simulink library "simulink"  (Simulink 6.0)
settings: Solver=ode45  SolverMode=SingleTasking  StartTime=0.0  StopTime=10.0  RelTol=1e-3
PostLoadFcn:
  | setsysloc(bdroot)
undefined symbols (not defined in the file or in its folder): DiscIntNeverNeededParam, getdatatypespecs, NumBits1, NumBits2, sfunxy, sigbuilder_block, slcm, Slope1, Slope2
libraries: simulink x82, eml_lib x1
(part 4 of 5)

== system simulink/Model Verification/Check  Dynamic Gap ==
  max : Inport  LatchInput=off
  min : Inport  Port=2  LatchInput=off
  u : Inport  Port=3  LatchInput=off
  Assertion : Assertion
      settings: CopyFcn=set_param(gcbh,'ShadowObject',get_param(get_param(gcbh,'Parent'),'Handle'));
  disjunction : Logic  Operator=OR
  max_relop : RelationalOperator  Operator=<  InputSameDT=on
  maxtype : DataTypeConversion  SaturateOnIntegerOverflow=on  RndMeth=Zero
  min_relop : RelationalOperator  Operator=<  InputSameDT=on
  mintype : DataTypeConversion  SaturateOnIntegerOverflow=on  RndMeth=Zero
  out : Terminator
  wires:
  max/1 -> maxtype/1
  min/1 -> mintype/1
  u/1 -> min_relop/1, max_relop/2
  disjunction/1 -> Assertion/1, out/1
  min_relop/1 -> disjunction/2
  max_relop/1 -> disjunction/1
  mintype/1 -> min_relop/2
  maxtype/1 -> max_relop/1

== system simulink/Model Verification/Check  Dynamic Range ==
  max : Inport  LatchInput=off
  min : Inport  Port=2  LatchInput=off
  u : Inport  Port=3  LatchInput=off
  Assertion : Assertion
      settings: CopyFcn=set_param(gcbh,'ShadowObject',get_param(get_param(gcbh,'Parent'),'Handle'));
  conjunction : Logic
  max_relop : RelationalOperator  Operator=<  InputSameDT=on
  maxtype : DataTypeConversion  SaturateOnIntegerOverflow=on  RndMeth=Zero
  min_relop : RelationalOperator  Operator=<  InputSameDT=on
  mintype : DataTypeConversion  SaturateOnIntegerOverflow=on  RndMeth=Zero
  out : Terminator
  wires:
  u/1 -> max_relop/1, min_relop/2
  min/1 -> mintype/1
  mintype/1 -> min_relop/1
  max/1 -> maxtype/1
  maxtype/1 -> max_relop/2
  min_relop/1 -> conjunction/1
  max_relop/1 -> conjunction/2
  conjunction/1 -> Assertion/1, out/1

== system simulink/Model Verification/Check  Static Gap ==
  u : Inport  LatchInput=off
  Assertion : Assertion
      settings: CopyFcn=set_param(gcbh,'ShadowObject',get_param(get_param(gcbh,'Parent'),'Handle'));
  disjunction : Logic  Operator=OR
  max_relop : RelationalOperator  Operator=<=  InputSameDT=on
  max_val : Constant  Value=max
  maxtype : DataTypeConversion  SaturateOnIntegerOverflow=on  RndMeth=Zero
  min_relop : RelationalOperator  Operator=<=  InputSameDT=on
  min_val : Constant  Value=min
  mintype : DataTypeConversion  SaturateOnIntegerOverflow=on  RndMeth=Zero
  out : Terminator
  wires:
  mintype/1 -> min_relop/2
  maxtype/1 -> max_relop/1
  min_val/1 -> mintype/1
  max_val/1 -> maxtype/1
  u/1 -> max_relop/2, min_relop/1
  max_relop/1 -> disjunction/1
  min_relop/1 -> disjunction/2
  disjunction/1 -> Assertion/1, out/1

== system simulink/Model Verification/Check  Static Range ==
  u : Inport  LatchInput=off
  Assertion : Assertion
      settings: CopyFcn=set_param(gcbh,'ShadowObject',get_param(get_param(gcbh,'Parent'),'Handle'));
  conjunction : Logic
  max_relop : RelationalOperator  Operator=<=  InputSameDT=on
  max_val : Constant  Value=max
  maxtype : DataTypeConversion  SaturateOnIntegerOverflow=on  RndMeth=Zero
  min_relop : RelationalOperator  Operator=<=  InputSameDT=on
  min_val : Constant  Value=min
  mintype : DataTypeConversion  SaturateOnIntegerOverflow=on  RndMeth=Zero
  out : Terminator
  wires:
  maxtype/1 -> max_relop/2
  mintype/1 -> min_relop/1
  conjunction/1 -> Assertion/1, out/1
  max_relop/1 -> conjunction/2
  min_relop/1 -> conjunction/1
  max_val/1 -> maxtype/1
  min_val/1 -> mintype/1
  u/1 -> max_relop/1, min_relop/2

== system simulink/Model Verification/Check Dynamic  Lower Bound ==
  min : Inport  LatchInput=off
  u : Inport  Port=2  LatchInput=off
  Assertion : Assertion
      settings: CopyFcn=set_param(gcbh,'ShadowObject',get_param(get_param(gcbh,'Parent'),'Handle'));
  min_relop : RelationalOperator  Operator=<  InputSameDT=on
  mintype : DataTypeConversion  SaturateOnIntegerOverflow=on  RndMeth=Zero
  out : Terminator
  wires:
  u/1 -> min_relop/2
  mintype/1 -> min_relop/1
  min/1 -> mintype/1
  min_relop/1 -> Assertion/1, out/1

== system simulink/Model Verification/Check Dynamic  Upper Bound ==
  max : Inport  LatchInput=off
  u : Inport  Port=2  LatchInput=off
  Assertion : Assertion
      settings: CopyFcn=set_param(gcbh,'ShadowObject',get_param(get_param(gcbh,'Parent'),'Handle'));
  max_relop : RelationalOperator  Operator=<  InputSameDT=on
  maxtype : DataTypeConversion  SaturateOnIntegerOverflow=on  RndMeth=Zero
  out : Terminator
  wires:
  u/1 -> max_relop/1
  max/1 -> maxtype/1
  maxtype/1 -> max_relop/2
  max_relop/1 -> Assertion/1, out/1

== system simulink/Model Verification/Check Input  Resolution ==
  u : Inport  LatchInput=off
  Assertion : Assertion
      settings: CopyFcn=set_param(gcbh,'ShadowObject',get_param(get_param(gcbh,'Parent'),'Handle'));
  dead_out : Terminator
  dead_resolution : Constant  Value=[1 1]
  dead_u : Constant
  fixed : Subsystem
  out : Terminator
  resolution : Constant  Value=resolution
  resolution_type : DataTypeConversion  SaturateOnIntegerOverflow=on  RndMeth=Zero
  steps : Subsystem
  wires:
  resolution/1 -> resolution_type/1
  u/1 -> steps/1(u)
  resolution_type/1 -> steps/2(resolution)
  steps/1(out) -> Assertion/1, out/1
  dead_u/1 -> fixed/1(u)
  dead_resolution/1 -> fixed/2(resolution)
  fixed/1(out) -> dead_out/1

== system simulink/Model Verification/Check Static  Lower Bound ==
  u : Inport  LatchInput=off
  Assertion : Assertion
      settings: CopyFcn=set_param(gcbh,'ShadowObject',get_param(get_param(gcbh,'Parent'),'Handle'));
  min_relop : RelationalOperator  Operator=<=  InputSameDT=on
  min_val : Constant  Value=min
  mintype : DataTypeConversion  SaturateOnIntegerOverflow=on  RndMeth=Zero
  out : Terminator
  wires:
  min_relop/1 -> Assertion/1, out/1
  u/1 -> min_relop/2
  min_val/1 -> mintype/1
  mintype/1 -> min_relop/1

== system simulink/Model Verification/Check Static  Upper Bound ==
  u : Inport  LatchInput=off
  Assertion : Assertion
      settings: CopyFcn=set_param(gcbh,'ShadowObject',get_param(get_param(gcbh,'Parent'),'Handle'));
  max_relop : RelationalOperator  Operator=<=  InputSameDT=on
  max_val : Constant  Value=max
  mintype : DataTypeConversion  SaturateOnIntegerOverflow=on  RndMeth=Zero
  out : Terminator
  wires:
  mintype/1 -> max_relop/2
  u/1 -> max_relop/1
  max_val/1 -> mintype/1
  max_relop/1 -> Assertion/1, out/1

== system simulink/Model-Wide Utilities/Block Support Table ==
  EmptySubsystem : Subsystem

== system simulink/Model-Wide Utilities/DocBlock ==
  EmptySubsystem : Subsystem

== system simulink/Model-Wide Utilities/Model Info ==
  EmptySubsystem : Subsystem

== system simulink/Model-Wide Utilities/Timed-Based Linearization ==
  Clock : Clock
      settings: Decimation=10
  Constant : Constant  Value=LinearizationTime
  Sum : Sum  Inputs=-+  SaturateOnIntegerOverflow=on  InputSameDT=on
  Triggered Linearization : Subsystem  Orientation=down  TreatAsAtomicUnit=on
  wires:
  Clock/1 -> Sum/2
  Constant/1 -> Sum/1
  Sum/1 -> Triggered Linearization/Trigger

== system simulink/Model-Wide Utilities/Trigger-Based Linearization ==
  Trigger : TriggerPort
  S-Function : S-Function  FunctionName=sfunlin  Parameters=name_,SampleTime

== system simulink/Ports & Subsystems/Atomic Subsystem ==
  In1 : Inport  LatchInput=off
  Out1 : Outport
  wires:
  In1/1 -> Out1/1

== system simulink/Ports & Subsystems/CodeReuseSubsystem ==
  In1 : Inport  LatchInput=off
  Out1 : Outport
  wires:
  In1/1 -> Out1/1

== system simulink/Ports & Subsystems/Configurable Subsystem ==

== system simulink/Ports & Subsystems/Enabled Subsystem ==
  In1 : Inport  LatchInput=off
  Enable : EnablePort
  Out1 : Outport
  wires:
  In1/1 -> Out1/1

== system simulink/Ports & Subsystems/Enabled and Triggered Subsystem ==
  In1 : Inport  LatchInput=off
  Enable : EnablePort
  Trigger : TriggerPort
  Out1 : Outport
  wires:
  In1/1 -> Out1/1

== system simulink/Ports & Subsystems/For Iterator Subsystem ==
  In1 : Inport  LatchInput=off
  For Iterator : ForIterator
  Out1 : Outport
  wires:
  In1/1 -> Out1/1

== system simulink/Ports & Subsystems/Function-Call Subsystem ==
  In1 : Inport  LatchInput=off
  function : TriggerPort  TriggerType=function-call
  Out1 : Outport
  wires:
  In1/1 -> Out1/1

== system simulink/Ports & Subsystems/If Action Subsystem ==
  In1 : Inport  LatchInput=off
  Action Port : ActionPort  ActionType=then
  Out1 : Outport
  wires:
  In1/1 -> Out1/1

== system simulink/Ports & Subsystems/Subsystem ==
  In1 : Inport  LatchInput=off
  Out1 : Outport
  wires:
  In1/1 -> Out1/1

== system simulink/Ports & Subsystems/Subsystem Examples ==
  Gain : Gain  SaturateOnIntegerOverflow=on

== system simulink/Ports & Subsystems/Switch Case Action Subsystem ==
  In1 : Inport  LatchInput=off
  Action Port : ActionPort  ActionType=case
  Out1 : Outport
  wires:
  In1/1 -> Out1/1

== system simulink/Ports & Subsystems/Triggered Subsystem ==
  In1 : Inport  LatchInput=off
  Trigger : TriggerPort
  Out1 : Outport
  wires:
  In1/1 -> Out1/1

== system simulink/Ports & Subsystems/While Iterator Subsystem ==
  In1 : Inport  LatchInput=off
  IC : Inport  Port=2  LatchInput=off
  While Iterator : WhileIterator
  Out1 : Outport
  wires:
  In1/1 -> Out1/1
  IC/1 -> While Iterator/2

== system simulink/Signal Attributes/Data Type Conversion Inherited ==
  DTS reference : Inport  LatchInput=off
  u : Inport  Port=2  LatchInput=off
  Conversion : DataTypeConversion  OutDataType=sint(16)  OutScaling=1  LockScale=on
  Data Type Prop : simulink/Signal Attributes/Data Type Propagation  PropDataType=sfix(16)  IfRefDouble=double  IfRefSingle=single  IsSigned=IsSigned1  NumBitsBase=NumBits1  NumBitsMult=1  NumBitsAdd=0  NumBitsAllowFinal=1:128  PropScaling=2^-10  ValuesUsedBestPrec=[5 -7]  SlopeBase=Slope1  SlopeMult=1  SlopeAdd=0  BiasBase=Bias1  BiasMult=1  BiasAdd=0
  y : Outport
  wires:
  u/1 -> Conversion/1
  DTS reference/1 -> Data Type Prop/1, Data Type Prop/2
  Conversion/1 -> y/1, Data Type Prop/3

== system simulink/Signal Attributes/Data Type Propagation Examples ==
  Gain : Gain  SaturateOnIntegerOverflow=on

== system simulink/Signal Attributes/Data Type Scaling Strip ==
  note: Force Scaling to be nominal,
      | slope == 1.0
      | bias == 0.0
  note: Gateway Out set to "auto"
      | which is similar to
      | "Inherit via back propagation"
  In : Inport  LatchInput=off
  FixPt Data Type Propagation : simulink/Signal Attributes/Data Type Propagation  PropDataType=sfix(16)  IfRefDouble=double  IfRefSingle=single  IsSigned=IsSigned1  NumBitsBase=NumBits1  NumBitsMult=1  NumBitsAdd=0  NumBitsAllowFinal=[8,16,32]  PropScalingMode=Specify via dialog  PropScaling=1  ValuesUsedBestPrec=[5 -7]  SlopeBase=Slope1  SlopeMult=0  SlopeAdd=1  BiasBase=Bias1  BiasMult=1  BiasAdd=0
  FixPt Gateway Out : DataTypeConversion  ConvertRealWorld=Stored Integer (SI)
  Out1 : Outport
  wires:
  In/1 -> FixPt Data Type Propagation/1, FixPt Data Type Propagation/2, FixPt Gateway Out/1
  FixPt Gateway Out/1 -> FixPt Data Type Propagation/3, Out1/1

== system simulink/Signal Routing/Environment Controller ==
  Sim : Inport  LatchInput=off
  RTW : Inport  Port=2  LatchInput=off
  Numerical Unity : SignalConversion  ConversionOutput=Contiguous copy
  Switch : Switch  DisableCoverage=on  Criteria=u2 ~= 0  ZeroCross=off  InputSameDT=on
  Switch Control : Constant  Value=switch_mode  OutDataTypeMode=boolean
  Out : Outport
  wires:
  Sim/1 -> Switch/1
  Switch Control/1 -> Switch/2
  Switch/1 -> Numerical Unity/1
  RTW/1 -> Switch/3
  Numerical Unity/1 -> Out/1

== system simulink/Signal Routing/Manual Switch ==
  1 : Inport  LatchInput=off
  2 : Inport  Port=2  LatchInput=off
  Environment Controller : simulink/Signal Routing/Environment Controller
  RTWValue : Constant  Value=boolean(1)  OutDataTypeMode=boolean
  SimValue : S-Function  FunctionName=sfun_manswitch  Parameters=boolean(1)
  Switch : Switch  Threshold=1
  Out1 : Outport
  wires:
  1/1 -> Switch/1
  2/1 -> Switch/3
  Switch/1 -> Out1/1
  SimValue/1 -> Environment Controller/1
  RTWValue/1 -> Environment Controller/2
  Environment Controller/1 -> Switch/2

== system simulink/Sinks/XY Graph ==
  x : Inport  LatchInput=off
  y : Inport  Port=2  LatchInput=off
  Data Type Conversion : DataTypeConversion  OutDataTypeMode=double
  Data Type Conversion1 : DataTypeConversion  OutDataTypeMode=double
  Mux : Mux  Inputs=2
  sfunxy : S-Function  FunctionName=sfunxy  Parameters=[xmin xmax ymin ymax], st
  wires:
  Mux/1 -> sfunxy/1
  x/1 -> Data Type Conversion/1
  y/1 -> Data Type Conversion1/1
  Data Type Conversion/1 -> Mux/1
  Data Type Conversion1/1 -> Mux/2

== system simulink/Sources/Band-Limited White Noise ==
  Output : Gain  Gain=[sqrt(Cov)]/[sqrt(Ts)]  SaturateOnIntegerOverflow=on
  White Noise : RandomNumber  DisableCoverage=on  Seed=seed  SampleTime=Ts
  Out1 : Outport
  wires:
  White Noise/1 -> Output/1
  Output/1 -> Out1/1

== system simulink/Sources/Chirp Signal ==
  note: freqSlope = deltaFreq/targetTime;
      | instantaneousFreq(t) = freqSlope*t + initialFreq;
      | intantaneousPhase(t) = integral(instFreq) = ...
      |       0.5*freqSlope*t^2 + initialFreq*t;
      | outputSignal(t) = sin(instantaneousPhase(t));
  Clock1 : Clock
      settings: DisableCoverage=on  Decimation=10
  Gain : Gain  DisableCoverage=on  Gain=0.5
  Output : Trigonometry
  Product : Product  DisableCoverage=on  Inputs=*/  SaturateOnIntegerOverflow=on  InputSameDT=on
  Product1 : Product  DisableCoverage=on  SaturateOnIntegerOverflow=on  InputSameDT=on
  Product2 : Product  DisableCoverage=on  SaturateOnIntegerOverflow=on  InputSameDT=on
  Sum : Sum  DisableCoverage=on  Inputs=|++  SaturateOnIntegerOverflow=on  InputSameDT=on
  deltaFreq : Constant  DisableCoverage=on  Value=2*pi*(f2-f1)
  initialFreq : Constant  DisableCoverage=on  Value=2*pi*f1
  targetTime : Constant  DisableCoverage=on  Value=T
  Out2 : Outport
  wires:
  deltaFreq/1 -> Product/1
  targetTime/1 -> Product/2
  Product/1 -> Gain/1
  Clock1/1 -> Product1/1, Product2/1
  Gain/1 -> Product1/2
  Product1/1 -> Sum/1
  initialFreq/1 -> Sum/2
  Sum/1 -> Product2/2
  Product2/1 -> Output/1
  Output/1 -> Out2/1

== system simulink/Sources/Counter Free-Running ==
  FixPt Data Type Propagation : simulink/Signal Attributes/Data Type Propagation  PropDataTypeMode=Specify via dialog  PropDataType=uint(NumBits)  IfRefDouble=double  IfRefSingle=single  IsSigned=IsSigned1 or IsSigned2  NumBitsBase=max([NumBits1 NumBits2])  NumBitsMult=1  NumBitsAdd=0  NumBitsAllowFinal=1:128  PropScalingMode=Specify via dialog  PropScaling=1  ValuesUsedBestPrec=[5 -7]  SlopeBase=min([Slope1 Slope2])  SlopeMult=1  SlopeAdd=0  BiasBase=Bias1  BiasMult=1  BiasAdd=0
  Force to be scalar : SignalSpecification  Orientation=left  Dimensions=1
  Increment Real World : simulink/Additional Math & Discrete/Additional Math: Increment - Decrement/Increment Real World
  Output : UnitDelay  X0=0.0  SampleTime=tsamp
  Wrap To Zero : simulink/Discontinuities/Wrap To Zero  Threshold=(2^(NumBits))-1
  y : Outport
  wires:
  Force to be scalar/1 -> Increment Real World/1
  Wrap To Zero/1 -> Output/1, FixPt Data Type Propagation/1, FixPt Data Type Propagation/3, FixPt Data Type Propagation/2
  Increment Real World/1 -> Wrap To Zero/1
  Output/1 -> Force to be scalar/1, y/1

== system simulink/Sources/Counter Limited ==
  Data Type Propagation : simulink/Signal Attributes/Data Type Propagation  PropDataTypeMode=Specify via dialog  PropDataType=uint(nbits)  IfRefDouble=double  IfRefSingle=single  IsSigned=IsSigned1 or IsSigned2  NumBitsBase=max([NumBits1 NumBits2])  NumBitsMult=1  NumBitsAdd=0  NumBitsAllowFinal=1:128  PropScalingMode=Specify via dialog  PropScaling=1  ValuesUsedBestPrec=[5 -7]  SlopeBase=min([Slope1 Slope2])  SlopeMult=1  SlopeAdd=0  BiasBase=Bias1  BiasMult=1  BiasAdd=0
  Force to be scalar : SignalSpecification  Orientation=left  Dimensions=1
  Increment Real World : simulink/Additional Math & Discrete/Additional Math: Increment - Decrement/Increment Real World
  Output : UnitDelay  X0=0.0  SampleTime=tsamp
  Wrap To Zero : simulink/Discontinuities/Wrap To Zero  Threshold=uplimit
  y : Outport
  wires:
  Force to be scalar/1 -> Increment Real World/1
  Increment Real World/1 -> Wrap To Zero/1
  Output/1 -> Force to be scalar/1, y/1
  Wrap To Zero/1 -> Data Type Propagation/3, Data Type Propagation/2, Data Type Propagation/1, Output/1

== system simulink/Sources/Ramp ==
  Clock : Clock
      settings: DisableCoverage=on  Decimation=10
  Constant : Constant  DisableCoverage=on  Value=start
  Constant1 : Constant  DisableCoverage=on  Value=X0
  Output : Sum  Inputs=|++  SaturateOnIntegerOverflow=on  InputSameDT=on
  Product : Product  DisableCoverage=on  SaturateOnIntegerOverflow=on  InputSameDT=on
  Step : Step  DisableCoverage=on  Time=start  After=slope  SampleTime=0
  Sum : Sum  DisableCoverage=on  Inputs=|+-  SaturateOnIntegerOverflow=on  InputSameDT=on
  Out1 : Outport
  wires:
  Step/1 -> Product/1
  Product/1 -> Output/1
  Constant1/1 -> Output/2
  Output/1 -> Out1/1
  Sum/1 -> Product/2
  Constant/1 -> Sum/2
  Clock/1 -> Sum/1

== system simulink/Sources/Repeating Sequence ==
  Clock : Clock
      settings: DisableCoverage=on  Decimation=10
  Fcn1 : Fcn  DisableCoverage=on  Expr=rem(u[1],period)
  Look-Up Table1 : Lookup  DisableCoverage=on  DialogController=Simulink.DDGSource  InputValues=rep_seq_t - min(rep_seq_t)  OutputValues=rep_seq_y  SaturateOnIntegerOverflow=on
  Output : SignalConversion  ConversionOutput=Contiguous copy
  Sum : Sum  DisableCoverage=on  Inputs=+-  SaturateOnIntegerOverflow=on  InputSameDT=on
  startTime : S-Function  DisableCoverage=on  FunctionName=sfun_tstart
  Out1 : Outport
  wires:
  Fcn1/1 -> Look-Up Table1/1
  Sum/1 -> Fcn1/1
  Clock/1 -> Sum/1
  startTime/1 -> Sum/2
  Look-Up Table1/1 -> Output/1
  Output/1 -> Out1/1

== system simulink/Sources/Repeating Sequence Interpolated ==
  Data Type Propagation : simulink/Signal Attributes/Data Type Propagation  PropDataType=sfix(16)  IfRefDouble=double  IfRefSingle=single  IsSigned=IsSigned2  NumBitsBase=NumBits2  NumBitsMult=1  NumBitsAdd=0  NumBitsAllowFinal=1:128  PropScaling=2^-10  ValuesUsedBestPrec=[5 -7]  SlopeBase=Slope2  SlopeMult=1  SlopeAdd=0  BiasBase=Bias2  BiasMult=1  BiasAdd=0
  Data Type Conversion : DataTypeConversion
  Force to be scalar : SignalSpecification  Dimensions=1
  LimitedCounter : simulink/Sources/Counter Limited  uplimit=nn  tsamp=tsamp
  Lookup : Lookup  DisableCoverage=on  DialogController=Simulink.DDGSource  InputValues=TimeValues  OutputValues=OutValues  LookUpMeth=Interpolation-Use End Values  OutDataTypeMode=Specify via dialog  OutDataType=OutDataType  OutScaling=OutScaling
  Output : SignalConversion  ConversionOutput=Contiguous copy
  Sample Time Math : simulink/Math Operations/Weighted Sample Time Math  TsampMathOp=*  weightValue=1.0  TsampMathImp=Offline Scaling Adjustment  DoSatur=off
  y : Outport
  wires:
  Output/1 -> y/1
  Lookup/1 -> Output/1, Data Type Propagation/1
  Force to be scalar/1 -> Data Type Conversion/1, Data Type Propagation/2
  LimitedCounter/1 -> Force to be scalar/1
  Sample Time Math/1 -> Lookup/1
  Data Type Conversion/1 -> Sample Time Math/1, Data Type Propagation/3

== system simulink/Sources/Repeating Sequence Stair ==
  Force to be scalar : SignalSpecification  Dimensions=1
  LimitedCounter : simulink/Sources/Counter Limited  uplimit=nn  tsamp=tsamp
  Out : SignalConversion  ConversionOutput=Contiguous copy
  Output : MultiPortSwitch  DisableCoverage=on  Inputs=1  zeroidx=on
  Vector : Constant  DisableCoverage=on  Value=OutValues  OutDataTypeMode=Specify via dialog  OutDataType=OutDataType  ConRadixGroup=Best Precision: Vector-wise  OutScaling=OutScaling
  y : Outport
  wires:
  Force to be scalar/1 -> Output/1
  Vector/1 -> Output/2
  LimitedCounter/1 -> Force to be scalar/1
  Output/1 -> Out/1
  Out/1 -> y/1

== system simulink/Sources/Signal Builder ==
  Demux : Demux  Tag=STV Demux  Outputs=1
  FromWs : FromWorkspace  Tag=STV FromWs  VariableName=tuvar  SampleTime=0  SigBuilderData=DataTag0
      SigBuilderData=|
      | channels.label = 'Signal 1'
      | channels.allXData = {[0 4 4 6 6 10]}
      | channels.allYData = {[0 0 1 1 0 0]}
      | dataSet.timeRange = [0 10]
      | dataSet.name = 'Group 1'
  Signal 1 : Outport  Tag=STV Outport
  wires:
  FromWs/1 -> Demux/1
  Demux/1 -> Signal 1/1

== system simulink/User-Defined Functions/S-Function Examples ==
  Gain : Gain  SaturateOnIntegerOverflow=on

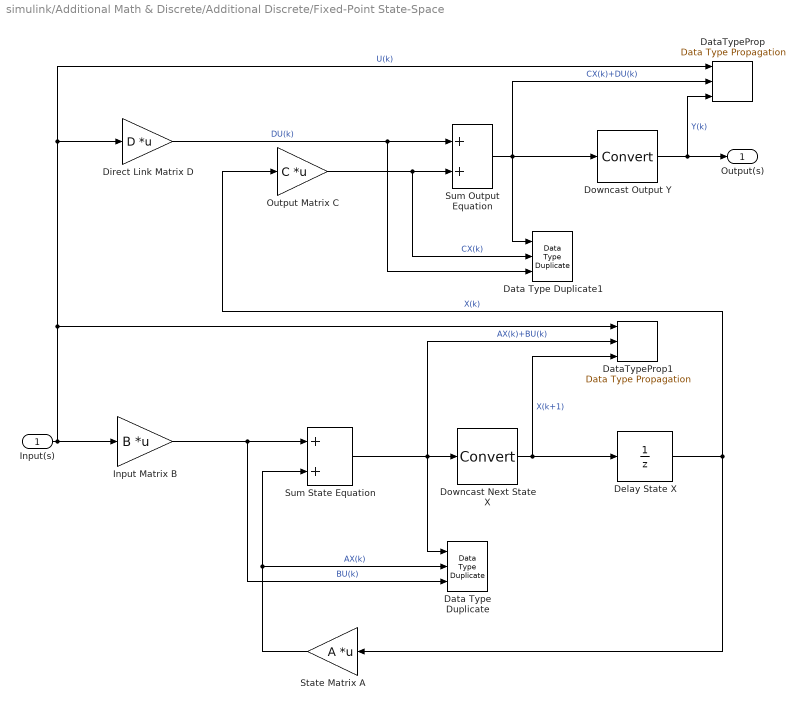
== system simulink/Additional Math & Discrete/Additional Discrete/Fixed-Point State-Space ==
  Input(s) : Inport  LatchInput=off
  Data Type Duplicate : simulink/Signal Attributes/Data Type Duplicate  NumInputPorts=3
  Data Type Duplicate1 : simulink/Signal Attributes/Data Type Duplicate  NumInputPorts=3
  DataTypeProp : simulink/Signal Attributes/Data Type Propagation  PropDataType=sfix(16)  IfRefDouble=double  IfRefSingle=single  IsSigned=IsSigned1 or IsSigned2  NumBitsBase=NumBits1  NumBitsMult=1  NumBitsAdd=0  NumBitsAllowFinal=1:128  PropScaling=2^-10  ValuesUsedBestPrec=[5 -7]  SlopeBase=PosRange2  SlopeMult=1  SlopeAdd=0  BiasBase=Bias2  BiasMult=1  BiasAdd=0
  DataTypeProp1 : simulink/Signal Attributes/Data Type Propagation  PropDataType=sfix(16)  IfRefDouble=double  IfRefSingle=single  IsSigned=IsSigned1 or IsSigned2  NumBitsBase=NumBits1  NumBitsMult=1  NumBitsAdd=0  NumBitsAllowFinal=1:128  PropScaling=2^-10  ValuesUsedBestPrec=[5 -7]  SlopeBase=PosRange2  SlopeMult=1  SlopeAdd=0  BiasBase=Bias2  BiasMult=1  BiasAdd=0
  Delay State X : UnitDelay  Description=Store in Global RAM  X0=X0  SampleTime=-1
      settings: AttributesFormatString=%<Description>
  Direct Link Matrix D : Gain  Description=Multiply in CPU  Gain=D  Multiplication=Matrix(K*u) (u vector)  ParameterDataType=sint(8)  ParameterScalingMode=Use specified scaling  ParameterScaling=1  OutDataType=sint(8)  OutScaling=1
      settings: AttributesFormatString=%<Description>
  Downcast Next State X : DataTypeConversion  Description=|  OutDataType=sint(8)  OutScaling=1
      | Reduce from CPU Size
      |  to Global RAM Size
      settings: AttributesFormatString=%<Description>
  Downcast Output Y : DataTypeConversion  Description=|  OutDataType=sint(8)  OutScaling=1
      | Reduce from CPU Size
      |  to Global RAM Size
      settings: AttributesFormatString=%<Description>
  Input Matrix B : Gain  Description=Multiply in CPU  Gain=B  Multiplication=Matrix(K*u) (u vector)  ParameterDataType=sint(8)  ParameterScalingMode=Use specified scaling  ParameterScaling=1  OutDataType=sint(8)  OutScaling=1
      settings: AttributesFormatString=%<Description>
  Output Matrix C : Gain  Description=Multiply in CPU  Gain=C  Multiplication=Matrix(K*u) (u vector)  ParameterDataType=sint(8)  ParameterScalingMode=Use specified scaling  ParameterScaling=1  OutDataType=sint(8)  OutScaling=1
      settings: AttributesFormatString=%<Description>
  State Matrix A : Gain  Description=Multiply in CPU  Orientation=left  Gain=A  Multiplication=Matrix(K*u) (u vector)  ParameterDataType=sint(8)  ParameterScalingMode=Use specified scaling  ParameterScaling=1  OutDataType=sint(8)  OutScaling=1
      settings: AttributesFormatString=%<Description>
  Sum Output Equation : Sum  Description=Add in CPU  OutDataTypeMode=Specify via dialog  OutDataType=InternalDataType  OutScaling=OutputEqScaling
      settings: AttributesFormatString=%<Description>
  Sum State Equation : Sum  Description=Add in CPU  OutDataTypeMode=Specify via dialog  OutDataType=InternalDataType  OutScaling=StateEqScaling
      settings: AttributesFormatString=%<Description>
  Output(s) : Outport  InitialOutput=0
  wires:
  Direct Link Matrix D/1 -> Data Type Duplicate1/3, Sum Output Equation/1  "DU(k)"
  Output Matrix C/1 -> Data Type Duplicate1/2, Sum Output Equation/2  "CX(k)"
  Sum Output Equation/1 -> DataTypeProp/2, Data Type Duplicate1/1, Downcast Output Y/1  "CX(k)+DU(k)"
  Downcast Output Y/1 -> DataTypeProp/3, Output(s)/1  "Y(k)"
  Delay State X/1 -> Output Matrix C/1, State Matrix A/1  "X(k)"
  Downcast Next State X/1 -> DataTypeProp1/3, Delay State X/1  "X(k+1)"
  Sum State Equation/1 -> DataTypeProp1/2, Data Type Duplicate/1, Downcast Next State X/1  "AX(k)+BU(k)"
  Input Matrix B/1 -> Data Type Duplicate/3, Sum State Equation/1  "BU(k)"
  Input(s)/1 -> DataTypeProp1/1, DataTypeProp/1, Direct Link Matrix D/1, Input Matrix B/1  "U(k)"
  State Matrix A/1 -> Data Type Duplicate/2, Sum State Equation/2  "AX(k)"

== system simulink/Additional Math & Discrete/Additional Discrete/Transfer Fcn Direct Form II ==
  Input : Inport  LatchInput=off
  DataTypeProp : simulink/Signal Attributes/Data Type Propagation  PropDataType=sfix(16)  IfRefDouble=double  IfRefSingle=single  IsSigned=IsSigned1 or IsSigned2  NumBitsBase=max([NumBits1 NumBits2])  NumBitsMult=1  NumBitsAdd=0  NumBitsAllowFinal=1:128  PropScaling=2^-10  ValuesUsedBestPrec=[5 -7]  SlopeBase=min([Slope1 Slope2])  SlopeMult=OutputSlopeMult  SlopeAdd=0  BiasBase=Bias1  BiasMult=0  BiasAdd=0
  DataTypeProp1 : simulink/Signal Attributes/Data Type Propagation  PropDataType=sfix(16)  IfRefDouble=double  IfRefSingle=single  IsSigned=IsSigned1 or IsSigned2  NumBitsBase=max([NumBits1 NumBits2])  NumBitsMult=1  NumBitsAdd=0  NumBitsAllowFinal=1:128  PropScaling=2^-10  ValuesUsedBestPrec=[5 -7]  SlopeBase=min([Slope1 Slope2])  SlopeMult=OutputSlopeMult2  SlopeAdd=0  BiasBase=Bias1  BiasMult=0  BiasAdd=0
  DenCoef : Gain  Orientation=left  Gain=DenCoefVec  Multiplication=Matrix(K*u) (u vector)  ParameterDataType=float('double')  ParameterScalingMode=Use specified scaling  ParameterScaling=1  OutScaling=2^-10
      settings: AttributesFormatString=|
      | Data Type and Scaling Inherited
      | with goal of NO Quantization Noise
      | Possible Overflow or Saturation
  Downcast : DataTypeConversion  Description=|  OutDataType=float('double')  OutScaling=1  LockScale=on
      | Reduce from CPU Size
      |  to Global RAM Size
      settings: AttributesFormatString=%<Description>
  Downcast1 : DataTypeConversion  Description=|  OutDataType=float('double')  OutScaling=1  LockScale=on
      | Reduce from CPU Size
      |  to Global RAM Size
      settings: AttributesFormatString=%<Description>
  Mux : Mux  Inputs=2
  NumCoef : Gain  Gain=NumCoefVec  Multiplication=Matrix(K*u) (u vector)  ParameterDataType=float('double')  ParameterScalingMode=Use specified scaling  ParameterScaling=1  OutScaling=2^-10
      settings: AttributesFormatString=|
      | Data Type and Scaling Inherited
      | with goal of NO Quantization Noise
      | Possible Overflow or Saturation
  Sum : Sum  Tag=S16 2^-10  Inputs=+-  OutDataType=sfix(32)  OutScaling=2^(-26)  LockScale=on
      settings: AttributesFormatString=|
      | Data Type and Scaling Inherited
      | with goal of NO Quantization Noise
      | Possible Overflow or Saturation
  Tapped Delay : simulink/Discrete/Tapped Delay  vinit=vinit  samptime=-1  NumDelays=-1  DelayOrder=Newest  includeCurrent=off
      settings: AttributesFormatString=|
      | Number of Taps
      | Inherited via Back Propagation
  Output : Outport
  wires:
  Sum/1 -> Downcast1/1
  DenCoef/1 -> Sum/2
  Input/1 -> DataTypeProp1/1, DataTypeProp1/2, DataTypeProp/2, DataTypeProp/1, Sum/1
  NumCoef/1 -> Downcast/1
  Tapped Delay/1 -> DenCoef/1, Mux/2
  Downcast1/1 -> DataTypeProp1/3, Mux/1, Tapped Delay/1
  Mux/1 -> NumCoef/1
  Downcast/1 -> Output/1, DataTypeProp/3

== system simulink/Additional Math & Discrete/Additional Discrete/Transfer Fcn Direct Form II Time Varying ==
  Input : Inport  LatchInput=off
  Num : Inport  Port=2  LatchInput=off
  Den No Lead : Inport  Port=3  LatchInput=off
  DataTypeProp : simulink/Signal Attributes/Data Type Propagation  PropDataType=sfix(16)  IfRefDouble=double  IfRefSingle=single  IsSigned=IsSigned1  NumBitsBase=NumBits1  NumBitsMult=1  NumBitsAdd=0  NumBitsAllowFinal=1:128  PropScaling=2^-10  ValuesUsedBestPrec=[5 -7]  SlopeBase=Slope1  SlopeMult=1  SlopeAdd=0  BiasBase=Bias1  BiasMult=1  BiasAdd=0
  DataTypeProp1 : simulink/Signal Attributes/Data Type Propagation  PropDataType=sfix(16)  IfRefDouble=double  IfRefSingle=single  IsSigned=IsSigned1  NumBitsBase=NumBits1  NumBitsMult=1  NumBitsAdd=0  NumBitsAllowFinal=1:128  PropScaling=2^-10  ValuesUsedBestPrec=[5 -7]  SlopeBase=Slope1  SlopeMult=2  SlopeAdd=0  BiasBase=Bias1  BiasMult=1  BiasAdd=0
  Dot1 : simulink/Math Operations/Dot Product  Orientation=left  OutDataType=sfix(16)  OutScaling=2^-10  DoSatur=off
      settings: AttributesFormatString=|
      | Data Type and Scaling Inherited
      | with goal of NO Quantization Noise
      | Possible Overflow or Saturation
  Dot2 : simulink/Math Operations/Dot Product  OutDataType=sfix(16)  OutScaling=2^-10  DoSatur=off
      settings: AttributesFormatString=|
      | Data Type and Scaling Inherited
      | with goal of NO Quantization Noise
      | Possible Overflow or Saturation
  Downcast : DataTypeConversion  Description=|  OutDataType=float('double')  OutScaling=1  LockScale=on
      | Reduce from CPU Size
      |  to Global RAM Size
      settings: AttributesFormatString=%<Description>
  Downcast1 : DataTypeConversion  Description=|  OutDataType=float('double')  OutScaling=1  LockScale=on
      | Reduce from CPU Size
      |  to Global RAM Size
      settings: AttributesFormatString=%<Description>
  Mux : Mux  Inputs=2
  Sum : Sum  Tag=S16 2^-10  Inputs=+-  OutDataType=sfix(32)  OutScaling=2^(-26)  LockScale=on
      settings: AttributesFormatString=|
      | Data Type and Scaling Inherited
      | with goal of NO Quantization Noise
      | Possible Overflow or Saturation
  Tapped Delay : simulink/Discrete/Tapped Delay  vinit=vinit  samptime=-1  NumDelays=-1  DelayOrder=Newest  includeCurrent=off
      settings: AttributesFormatString=|
      | Number of Taps
      | Inherited via Back Propagation
  Output : Outport
  wires:
  Den No Lead/1 -> Dot1/2
  Num/1 -> Dot2/2
  Downcast/1 -> DataTypeProp/3, Output/1
  Mux/1 -> Dot2/1
  Downcast1/1 -> DataTypeProp1/3, Tapped Delay/1, Mux/1
  Tapped Delay/1 -> Dot1/1, Mux/2
  Dot2/1 -> Downcast/1
  Input/1 -> Sum/1, DataTypeProp1/2, DataTypeProp1/1, DataTypeProp/2, DataTypeProp/1
  Dot1/1 -> Sum/2
  Sum/1 -> Downcast1/1

== system simulink/Additional Math & Discrete/Additional Discrete/Unit Delay Enabled ==
  u : Inport  LatchInput=off
  E : Inport  Port=2  LatchInput=off
  Enable : Switch  Criteria=u2 ~= 0  ZeroCross=off
  FixPt Data Type Duplicate1 : simulink/Signal Attributes/Data Type Duplicate  NumInputPorts=3
  FixPt Unit Delay1 : UnitDelay  X0=vinit  SampleTime=tsamp
  y : Outport
  wires:
  E/1 -> Enable/2  "Enable"
  u/1 -> FixPt Data Type Duplicate1/3, Enable/1
  Enable/1 -> FixPt Unit Delay1/1, FixPt Data Type Duplicate1/2  "Xnew"
  FixPt Unit Delay1/1 -> y/1, Enable/3, FixPt Data Type Duplicate1/1  "Xold"

== system simulink/Additional Math & Discrete/Additional Discrete/Unit Delay Enabled External IC ==
  u : Inport  LatchInput=off
  E : Inport  Port=2  LatchInput=off
  IC : Inport  Port=3  LatchInput=off
  Enable : Switch  Criteria=u2 ~= 0  ZeroCross=off
  FixPt Data Type Duplicate1 : simulink/Signal Attributes/Data Type Duplicate  NumInputPorts=4
  Unit Delay External IC : simulink/Additional Math & Discrete/Additional Discrete/Unit Delay External IC  tsamp=tsamp
  y : Outport
  wires:
  E/1 -> Enable/2  "Enable"
  IC/1 -> FixPt Data Type Duplicate1/3, Unit Delay External IC/2  "Initial Value"
  u/1 -> FixPt Data Type Duplicate1/4, Enable/1
  Enable/1 -> FixPt Data Type Duplicate1/2, Unit Delay External IC/1  "Xnew"
  Unit Delay External IC/1 -> y/1, Enable/3, FixPt Data Type Duplicate1/1

== system simulink/Additional Math & Discrete/Additional Discrete/Unit Delay Enabled Resettable ==
  u : Inport  LatchInput=off
  E : Inport  Port=2  LatchInput=off
  R : Inport  Port=3  LatchInput=off
  Enable : Switch  Criteria=u2 ~= 0  ZeroCross=off
  FixPt Data Type Duplicate2 : simulink/Signal Attributes/Data Type Duplicate  NumInputPorts=3
  Unit Delay Resettable : simulink/Additional Math & Discrete/Additional Discrete/Unit Delay Resettable  vinit=vinit  tsamp=-1
  y : Outport
  wires:
  E/1 -> Enable/2  "Enable"
  u/1 -> Enable/1, FixPt Data Type Duplicate2/3
  Enable/1 -> FixPt Data Type Duplicate2/2, Unit Delay Resettable/1  "Xnew"
  Unit Delay Resettable/1 -> FixPt Data Type Duplicate2/1, Enable/3, y/1
  R/1 -> Unit Delay Resettable/2  "Reset"

== system simulink/Additional Math & Discrete/Additional Discrete/Unit Delay Enabled Resettable External IC ==
  u : Inport  LatchInput=off
  E : Inport  Port=2  LatchInput=off
  R : Inport  Port=3  LatchInput=off
  IC : Inport  Port=4  LatchInput=off
  Enable : Switch  Criteria=u2 ~= 0  ZeroCross=off
  FixPt Data Type Duplicate1 : simulink/Signal Attributes/Data Type Duplicate  NumInputPorts=4
  Unit Delay Resettable External IC : simulink/Additional Math & Discrete/Additional Discrete/Unit Delay Resettable External IC  tsamp=tsamp
  y : Outport
  wires:
  Unit Delay Resettable External IC/1 -> y/1, Enable/3, FixPt Data Type Duplicate1/1
  R/1 -> Unit Delay Resettable External IC/2  "Reset"
  Enable/1 -> Unit Delay Resettable External IC/1, FixPt Data Type Duplicate1/3
  u/1 -> Enable/1, FixPt Data Type Duplicate1/4
  IC/1 -> Unit Delay Resettable External IC/3, FixPt Data Type Duplicate1/2  "Initial Value"
  E/1 -> Enable/2  "Enable"

== system simulink/Additional Math & Discrete/Additional Discrete/Unit Delay External IC ==
  u : Inport  LatchInput=off
  IC : Inport  Port=2  LatchInput=off
  FixPt Constant : Constant  Value=0  OutDataTypeMode=Specify via dialog  OutDataType=uint(8)  OutScaling=1
  FixPt Data Type Duplicate1 : simulink/Signal Attributes/Data Type Duplicate  NumInputPorts=3
  FixPt Unit Delay1 : UnitDelay  X0=0.0  SampleTime=tsamp
  FixPt Unit Delay2 : UnitDelay  X0=1  SampleTime=tsamp
  Init : Switch  Criteria=u2 ~= 0  ZeroCross=off
  y : Outport
  wires:
  FixPt Unit Delay1/1 -> Init/3  "Xold"
  Init/1 -> y/1, FixPt Data Type Duplicate1/1
  FixPt Unit Delay2/1 -> Init/2
  FixPt Constant/1 -> FixPt Unit Delay2/1
  u/1 -> FixPt Unit Delay1/1, FixPt Data Type Duplicate1/2  "Xnew"
  IC/1 -> Init/1, FixPt Data Type Duplicate1/3  "Initial Value"

== system simulink/Additional Math & Discrete/Additional Discrete/Unit Delay Resettable ==
  u : Inport  LatchInput=off
  R : Inport  Port=2  LatchInput=off
  FixPt Constant : Constant  Value=0  OutDataTypeMode=Specify via dialog  OutDataType=uint(8)  OutScaling=1
  FixPt Data Type Duplicate1 : simulink/Signal Attributes/Data Type Duplicate  NumInputPorts=4
  FixPt Logical Operator : Logic  Operator=OR  AllPortsSameDT=off  OutDataTypeMode=Specify via dialog
  FixPt Unit Delay1 : UnitDelay  X0=vinit  SampleTime=tsamp
  FixPt Unit Delay2 : UnitDelay  X0=1  SampleTime=tsamp
  Init : Switch  Criteria=u2 ~= 0  ZeroCross=off
  Initial Condition : Constant  Value=vinit  OutDataType=uint(8)  OutScaling=1
  Reset : Switch  Criteria=u2 ~= 0  ZeroCross=off
  y : Outport
  wires:
  Initial Condition/1 -> Reset/1, Init/1, FixPt Data Type Duplicate1/3  "Initial Value"
  u/1 -> FixPt Data Type Duplicate1/4, Reset/3
  Reset/1 -> FixPt Data Type Duplicate1/2, FixPt Unit Delay1/1  "Xnew"
  R/1 -> Reset/2, FixPt Logical Operator/1  "Reset"
  FixPt Constant/1 -> FixPt Unit Delay2/1
  FixPt Unit Delay2/1 -> FixPt Logical Operator/2
  Init/1 -> FixPt Data Type Duplicate1/1, y/1
  FixPt Unit Delay1/1 -> Init/3  "Xold"
  FixPt Logical Operator/1 -> Init/2

== system simulink/Additional Math & Discrete/Additional Discrete/Unit Delay Resettable External IC ==
  u : Inport  LatchInput=off
  R : Inport  Port=2  LatchInput=off
  IC : Inport  Port=3  LatchInput=off
  FixPt Constant : Constant  Value=0  OutDataTypeMode=Specify via dialog  OutDataType=uint(8)  OutScaling=1
  FixPt Data Type Duplicate1 : simulink/Signal Attributes/Data Type Duplicate  NumInputPorts=4
  FixPt Logical Operator : Logic  Operator=OR  AllPortsSameDT=off  OutDataTypeMode=Specify via dialog
  FixPt Unit Delay1 : UnitDelay  X0=0.0  SampleTime=tsamp
  FixPt Unit Delay2 : UnitDelay  X0=1  SampleTime=tsamp
  Init : Switch  Criteria=u2 ~= 0  ZeroCross=off
  Reset : Switch  Criteria=u2 ~= 0  ZeroCross=off
  y : Outport
  wires:
  IC/1 -> Reset/1, Init/1, FixPt Data Type Duplicate1/3  "Initial Value"
  u/1 -> FixPt Data Type Duplicate1/4, Reset/3
  Reset/1 -> FixPt Data Type Duplicate1/2, FixPt Unit Delay1/1  "Xnew"
  R/1 -> Reset/2, FixPt Logical Operator/1  "Reset"
  FixPt Constant/1 -> FixPt Unit Delay2/1
  FixPt Unit Delay2/1 -> FixPt Logical Operator/2
  Init/1 -> FixPt Data Type Duplicate1/1, y/1
  FixPt Unit Delay1/1 -> Init/3  "Xold"
  FixPt Logical Operator/1 -> Init/2

== system simulink/Additional Math & Discrete/Additional Discrete/Unit Delay With Preview Enabled ==
  u : Inport  LatchInput=off
  E : Inport  Port=2  LatchInput=off
  Enable : Switch  Criteria=u2 ~= 0  ZeroCross=off
  FixPt Data Type Duplicate1 : simulink/Signal Attributes/Data Type Duplicate  NumInputPorts=3
  FixPt Unit Delay1 : UnitDelay  X0=vinit  SampleTime=tsamp
  y : Outport
  x : Outport  Port=2
  wires:
  FixPt Unit Delay1/1 -> FixPt Data Type Duplicate1/1, Enable/3, x/1  "Xold"
  Enable/1 -> FixPt Data Type Duplicate1/2, FixPt Unit Delay1/1, y/1  "Xnew"
  u/1 -> Enable/1, FixPt Data Type Duplicate1/3
  E/1 -> Enable/2  "Enable"

== system simulink/Additional Math & Discrete/Additional Discrete/Unit Delay With Preview Enabled Resettable ==
  u : Inport  LatchInput=off
  E : Inport  Port=2  LatchInput=off
  R : Inport  Port=3  LatchInput=off
  Enable : Switch  Criteria=u2 ~= 0  ZeroCross=off
  FixPt Data Type Duplicate2 : simulink/Signal Attributes/Data Type Duplicate  NumInputPorts=5
  FixPt Unit Delay1 : UnitDelay  X0=vinit  SampleTime=tsamp
  Initial Condition : Constant  Value=vinit  OutDataType=uint(8)  OutScaling=1
  Reset : Switch  Criteria=u2 ~= 0  InputSameDT=on
  y : Outport
  x : Outport  Port=2
  wires:
  E/1 -> Enable/2  "Enable"
  Initial Condition/1 -> FixPt Data Type Duplicate2/3, Reset/1  "Reset Value"
  u/1 -> FixPt Data Type Duplicate2/5, Enable/1
  Enable/1 -> FixPt Data Type Duplicate2/4, Reset/3
  FixPt Unit Delay1/1 -> x/1, Enable/3, FixPt Data Type Duplicate2/1  "Xold"
  Reset/1 -> y/1, FixPt Data Type Duplicate2/2, FixPt Unit Delay1/1  "Xnew"
  R/1 -> Reset/2  "Reset"

== system simulink/Additional Math & Discrete/Additional Discrete/Unit Delay With Preview Enabled Resettable External RV ==
  u : Inport  LatchInput=off
  E : Inport  Port=2  LatchInput=off
  R : Inport  Port=3  LatchInput=off
  V : Inport  Port=4  LatchInput=off
  Enable : Switch  Criteria=u2 ~= 0  ZeroCross=off
  FixPt Data Type Duplicate2 : simulink/Signal Attributes/Data Type Duplicate  NumInputPorts=5
  FixPt Unit Delay1 : UnitDelay  X0=vinit  SampleTime=tsamp
  Reset : Switch  Criteria=u2 ~= 0  InputSameDT=on
  y1 : Outport
  y2 : Outport  Port=2
  wires:
  R/1 -> Reset/2  "Reset"
  Reset/1 -> FixPt Unit Delay1/1, FixPt Data Type Duplicate2/2, y1/1  "Xnew"
  FixPt Unit Delay1/1 -> FixPt Data Type Duplicate2/1, Enable/3, y2/1  "Xold"
  Enable/1 -> Reset/3, FixPt Data Type Duplicate2/4
  u/1 -> Enable/1, FixPt Data Type Duplicate2/5  "Input"
  V/1 -> Reset/1, FixPt Data Type Duplicate2/3  "Reset Value"
  E/1 -> Enable/2  "Enable"

== system simulink/Additional Math & Discrete/Additional Discrete/Unit Delay With Preview Resettable ==
  u : Inport  LatchInput=off
  R : Inport  Port=2  LatchInput=off
  FixPt Data Type Duplicate2 : simulink/Signal Attributes/Data Type Duplicate  NumInputPorts=4
  FixPt Unit Delay1 : UnitDelay  X0=vinit  SampleTime=tsamp
  Initial Condition : Constant  Value=vinit  OutDataType=uint(8)  OutScaling=1
  Reset : Switch  Criteria=u2 ~= 0  ZeroCross=off
  y : Outport
  x : Outport  Port=2
  wires:
  Initial Condition/1 -> FixPt Data Type Duplicate2/3, Reset/1  "Reset Value"
  u/1 -> Reset/3, FixPt Data Type Duplicate2/4
  FixPt Unit Delay1/1 -> x/1, FixPt Data Type Duplicate2/1  "Xold"
  Reset/1 -> y/1, FixPt Data Type Duplicate2/2, FixPt Unit Delay1/1  "Xnew"
  R/1 -> Reset/2  "Reset"

== system simulink/Additional Math & Discrete/Additional Discrete/Unit Delay With Preview Resettable External RV ==
  u : Inport  LatchInput=off
  R : Inport  Port=2  LatchInput=off
  RV : Inport  Port=3  LatchInput=off
  FixPt Data Type Duplicate2 : simulink/Signal Attributes/Data Type Duplicate  NumInputPorts=4
  FixPt Unit Delay1 : UnitDelay  X0=vinit  SampleTime=tsamp
  Reset : Switch  Criteria=u2 ~= 0  ZeroCross=off
  y : Outport
  x : Outport  Port=2
  wires:
  RV/1 -> FixPt Data Type Duplicate2/3, Reset/1  "Reset Value"
  FixPt Unit Delay1/1 -> x/1, FixPt Data Type Duplicate2/1  "Xold"
  Reset/1 -> y/1, FixPt Data Type Duplicate2/2, FixPt Unit Delay1/1  "Xnew"
  R/1 -> Reset/2  "Reset"
  u/1 -> Reset/3, FixPt Data Type Duplicate2/4

== system simulink/Additional Math & Discrete/Additional Math: Increment - Decrement/Decrement Real World ==
  u : Inport  LatchInput=off
  FixPt Constant : Constant  ConRadixGroup=Best Precision: Vector-wise  OutScaling=2^-14
  FixPt Data Type Duplicate : simulink/Signal Attributes/Data Type Duplicate  NumInputPorts=3
  FixPt Sum1 : Sum  Inputs=+-  OutDataType=uint(4)  OutScaling=1  InputSameDT=on  LockScale=on
  y : Outport
  wires:
  FixPt Sum1/1 -> y/1, FixPt Data Type Duplicate/1
  FixPt Constant/1 -> FixPt Sum1/2, FixPt Data Type Duplicate/3
  u/1 -> FixPt Sum1/1, FixPt Data Type Duplicate/2

== system simulink/Additional Math & Discrete/Additional Math: Increment - Decrement/Decrement Stored Integer ==
  u : Inport  LatchInput=off
  FixPt Constant : Constant  ConRadixGroup=Best Precision: Vector-wise  OutScaling=2^-14
  FixPt Data Type Duplicate : simulink/Signal Attributes/Data Type Duplicate  NumInputPorts=3
  FixPt Data Type Propagation : simulink/Signal Attributes/Data Type Propagation  PropDataType=sfix(16)  IfRefDouble=double  IfRefSingle=single  IsSigned=IsSigned1  NumBitsBase=NumBits1  NumBitsMult=1  NumBitsAdd=0  NumBitsAllowFinal=1:128  PropScaling=2^-10  ValuesUsedBestPrec=[5 -7]  SlopeBase=Slope1  SlopeMult=0  SlopeAdd=1  BiasBase=Bias1  BiasMult=0  BiasAdd=0
  FixPt Gateway In : DataTypeConversion  OutScaling=2^-10  ConvertRealWorld=Stored Integer (SI)
  FixPt Sum1 : Sum  Inputs=+-  OutDataType=uint(4)  OutScaling=1  InputSameDT=on  LockScale=on
  y : Outport
  wires:
  u/1 -> FixPt Data Type Duplicate/2, FixPt Sum1/1
  FixPt Constant/1 -> FixPt Gateway In/1, FixPt Data Type Propagation/3
  FixPt Sum1/1 -> FixPt Data Type Duplicate/1, y/1
  FixPt Gateway In/1 -> FixPt Data Type Duplicate/3, FixPt Sum1/2, FixPt Data Type Propagation/1, FixPt Data Type Propagation/2

== system simulink/Additional Math & Discrete/Additional Math: Increment - Decrement/Decrement To Zero ==
  u : Inport  LatchInput=off
  FixPt Constant : Constant  ConRadixGroup=Best Precision: Vector-wise  OutScaling=2^-14
  FixPt Data Type Duplicate : simulink/Signal Attributes/Data Type Duplicate  NumInputPorts=5
  FixPt Relational Operator3 : RelationalOperator  Operator=>  LogicOutDataTypeMode=Specify via dialog  ZeroCross=off
  FixPt Sum1 : Sum  Inputs=+-  OutDataType=uint(4)  OutScaling=1  LockScale=on
  FixPt Switch4 : Switch  Threshold=1  ZeroCross=off
  Ground1 : Ground
  y : Outport
  wires:
  FixPt Switch4/1 -> FixPt Data Type Duplicate/1, y/1
  Ground1/1 -> FixPt Data Type Duplicate/2, FixPt Switch4/3
  FixPt Relational Operator3/1 -> FixPt Switch4/2
  u/1 -> FixPt Relational Operator3/1, FixPt Data Type Duplicate/4, FixPt Sum1/1
  FixPt Constant/1 -> FixPt Relational Operator3/2, FixPt Data Type Duplicate/5, FixPt Sum1/2
  FixPt Sum1/1 -> FixPt Switch4/1, FixPt Data Type Duplicate/3

== system simulink/Additional Math & Discrete/Additional Math: Increment - Decrement/Decrement Time To Zero ==
  u : Inport  LatchInput=off
  FixPt Data Type Duplicate : simulink/Signal Attributes/Data Type Duplicate  NumInputPorts=5
  FixPt Relational Operator3 : RelationalOperator  Operator=>  LogicOutDataTypeMode=Specify via dialog  ZeroCross=off
  FixPt Sample Time Math : simulink/Signal Attributes/Weighted Sample Time  TsampMathOp=Ts Only  weightValue=1.0  TsampMathImp=Online Calculations  DoSatur=off
  FixPt Sum1 : Sum  Inputs=+-  OutDataType=uint(4)  OutScaling=1  LockScale=on
  FixPt Switch4 : Switch  Threshold=1  ZeroCross=off
  Ground1 : Ground
  y : Outport
  wires:
  FixPt Switch4/1 -> FixPt Data Type Duplicate/1, y/1
  Ground1/1 -> FixPt Data Type Duplicate/2, FixPt Switch4/3
  FixPt Relational Operator3/1 -> FixPt Switch4/2
  u/1 -> FixPt Relational Operator3/1, FixPt Data Type Duplicate/4, FixPt Sum1/1, FixPt Sample Time Math/1
  FixPt Sample Time Math/1 -> FixPt Relational Operator3/2, FixPt Data Type Duplicate/5, FixPt Sum1/2
  FixPt Sum1/1 -> FixPt Switch4/1, FixPt Data Type Duplicate/3

== system simulink/Additional Math & Discrete/Additional Math: Increment - Decrement/Increment Real World ==
  u : Inport  LatchInput=off
  FixPt Constant : Constant  ConRadixGroup=Best Precision: Vector-wise  OutScaling=2^-14
  FixPt Data Type Duplicate : simulink/Signal Attributes/Data Type Duplicate  NumInputPorts=3
  FixPt Sum1 : Sum  OutDataType=uint(4)  OutScaling=1  InputSameDT=on  LockScale=on
  y : Outport
  wires:
  u/1 -> FixPt Data Type Duplicate/2, FixPt Sum1/1
  FixPt Constant/1 -> FixPt Data Type Duplicate/3, FixPt Sum1/2
  FixPt Sum1/1 -> FixPt Data Type Duplicate/1, y/1

== system simulink/Additional Math & Discrete/Additional Math: Increment - Decrement/Increment Stored Integer ==
  u : Inport  LatchInput=off
  FixPt Constant : Constant  ConRadixGroup=Best Precision: Vector-wise  OutScaling=2^-14
  FixPt Data Type Duplicate : simulink/Signal Attributes/Data Type Duplicate  NumInputPorts=3
  FixPt Data Type Propagation : simulink/Signal Attributes/Data Type Propagation  PropDataType=sfix(16)  IfRefDouble=double  IfRefSingle=single  IsSigned=IsSigned1  NumBitsBase=NumBits1  NumBitsMult=1  NumBitsAdd=0  NumBitsAllowFinal=1:128  PropScaling=2^-10  ValuesUsedBestPrec=[5 -7]  SlopeBase=Slope1  SlopeMult=0  SlopeAdd=1  BiasBase=Bias1  BiasMult=0  BiasAdd=0
  FixPt Gateway In : DataTypeConversion  OutScaling=2^-10  ConvertRealWorld=Stored Integer (SI)
  FixPt Sum1 : Sum  OutDataType=uint(4)  OutScaling=1  InputSameDT=on  LockScale=on
  y : Outport
  wires:
  FixPt Gateway In/1 -> FixPt Data Type Propagation/2, FixPt Data Type Propagation/1, FixPt Sum1/2, FixPt Data Type Duplicate/3
  FixPt Sum1/1 -> y/1, FixPt Data Type Duplicate/1
  FixPt Constant/1 -> FixPt Data Type Propagation/3, FixPt Gateway In/1
  u/1 -> FixPt Sum1/1, FixPt Data Type Duplicate/2

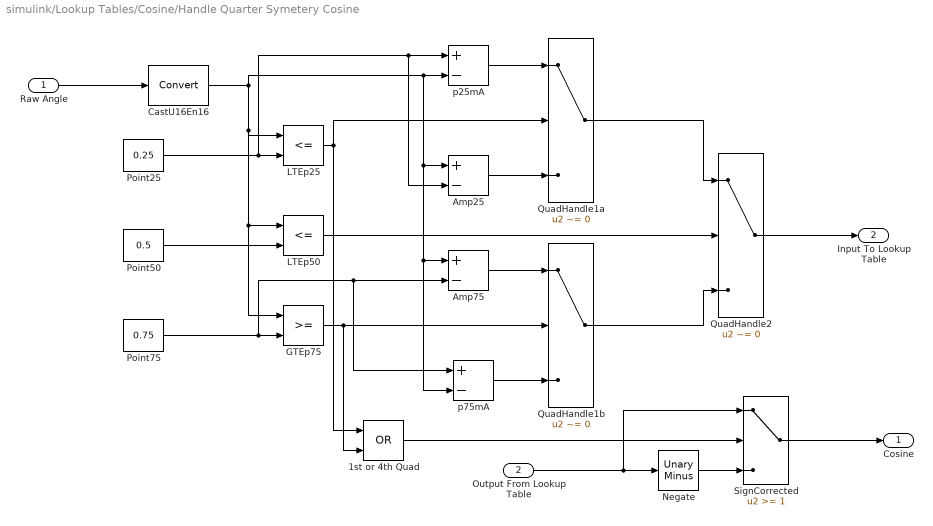
== system simulink/Lookup Tables/Cosine/Handle Quarter Symetery Cosine ==
  Raw Angle : Inport  LatchInput=off
  Output From Lookup Table : Inport  Port=2  LatchInput=off
  1st or 4th Quad : Logic  Operator=OR  AllPortsSameDT=off  OutDataTypeMode=Specify via dialog
  Amp25 : Sum  Inputs=+-  OutDataType=uint(8)  OutScaling=1  LockScale=on
  Amp75 : Sum  Inputs=+-  OutDataType=uint(8)  OutScaling=1  LockScale=on
  CastU16En16 : DataTypeConversion  OutDataTypeMode=Specify via dialog  OutDataType=ufix(16)  OutScaling=2^-16  LockScale=on
  GTEp75 : RelationalOperator  LogicOutDataTypeMode=Specify via dialog  ZeroCross=off
  LTEp25 : RelationalOperator  Operator=<=  LogicOutDataTypeMode=Specify via dialog  ZeroCross=off
  LTEp50 : RelationalOperator  Operator=<=  LogicOutDataTypeMode=Specify via dialog  ZeroCross=off
  Negate : simulink/Math Operations/Unary Minus  DoSatur=off
  Point25 : Constant  Value=0.25  OutDataTypeMode=Specify via dialog  OutDataType=ufix(16)  OutScaling=2^-16
  Point50 : Constant  Value=0.5  OutDataTypeMode=Specify via dialog  OutDataType=ufix(16)  OutScaling=2^-16
  Point75 : Constant  Value=0.75  OutDataTypeMode=Specify via dialog  OutDataType=ufix(16)  OutScaling=2^-16
  QuadHandle1a : Switch  Criteria=u2 ~= 0  ZeroCross=off
  QuadHandle1b : Switch  Criteria=u2 ~= 0  ZeroCross=off
  QuadHandle2 : Switch  Criteria=u2 ~= 0  ZeroCross=off
  SignCorrected : Switch  Threshold=1  ZeroCross=off
  p25mA : Sum  Inputs=+-  OutDataType=uint(8)  OutScaling=1  LockScale=on
  p75mA : Sum  Inputs=+-  OutDataType=uint(8)  OutScaling=1  LockScale=on
  Cosine : Outport
  Input To Lookup Table : Outport  Port=2
  wires:
  1st or 4th Quad/1 -> SignCorrected/2
  QuadHandle2/1 -> Input To Lookup Table/1
  QuadHandle1b/1 -> QuadHandle2/3
  QuadHandle1a/1 -> QuadHandle2/1
  GTEp75/1 -> 1st or 4th Quad/2, QuadHandle1b/2
  p75mA/1 -> QuadHandle1b/3
  Amp75/1 -> QuadHandle1b/1
  LTEp25/1 -> 1st or 4th Quad/1, QuadHandle1a/2
  LTEp50/1 -> QuadHandle2/2
  Amp25/1 -> QuadHandle1a/3
  Point50/1 -> LTEp50/2
  p25mA/1 -> QuadHandle1a/1
  Point75/1 -> p75mA/1, Amp75/2, GTEp75/2
  CastU16En16/1 -> p75mA/2, Amp75/1, Amp25/1, p25mA/2, GTEp75/1, LTEp50/1, LTEp25/1
  Negate/1 -> SignCorrected/3
  SignCorrected/1 -> Cosine/1
  Output From Lookup Table/1 -> SignCorrected/1, Negate/1
  Point25/1 -> Amp25/2, p25mA/1, LTEp25/2
  Raw Angle/1 -> CastU16En16/1
